simulink model "sim_aut_dual_scen"  (R2025b)
settings: Solver=ode45  StartTime=0.0  StopTime=Tfin  FixedStep=1e-3  MaxStep=1e-2  MinStep=1e-3  RelTol=5e-3
values from neighbouring files (symbols this model uses):
  bp = [-1.25 -1.19897959184 -1.14795918367 -1.09693877551 -1.04591836735 -0.994897959184 -0.94387755102 -0.892857142857 -0.841836734694 -0.790816326531 -0.739795918367 -0.688775510204 ... (50 elements, 1x50)]    [tire_model.mat]
  C1 = 2.7e4    (= 27000)    [main.m]    (also in model.m)
  C2 = 2e4    (= 20000)    [main.m]    (also in model.m)
  Jz = 4000    [main.m]    (also in model.m)
  K = nmpc_design_st2(par,2)    [main.m]
  l1 = 1.2    [main.m]    (also in model.m)
  l2 = 1.6    [main.m]    (also in model.m)
  m = 1575    [main.m]    (also in model.m)
  Np = round(vx_ref*K.Tp/mean(ds))    [main.m]
  pacf = [2550.90487699 2674.70463742 2810.77279096 2960.97362657 3127.55760929 3313.26346728 3521.4532226 3756.29269015 4022.99538347 4328.15571957 4680.20907939 5090.07319782 ... (50 elements, 1x50)]    [tire_model.mat]
  pacr = [2550.90487699 2674.70463742 2810.77279096 2960.97362657 3127.55760929 3313.26346728 3521.4532226 3756.29269015 4022.99538347 4328.15571957 4680.20907939 5090.07319782 ... (50 elements, 1x50)]    [tire_model.mat]
  psi = x(3)    [model.m]
  psir = [atan2(diff(Yr),diff(Xr));0]    [main.m]
  refPoses = [Xr,Yr,psir]    [main.m]
  Ts = 0.05    [main.m]
  ze0 = [X0;Y0;psi0;vx0;vy0;wpsi0]    [main.m]
undefined symbols (not defined in the file or in its folder): aMode, plot_ref, x_o
libraries: autolibsharedcommon x11, autolibshared x5, autolibpowerinfoutils x2, autolibutils x2, sharedtransform x2, simulink x1, drivingscenarioandsensors x1
(part 3 of 4)

== system sim_aut_dual_scen/vehicle/dual-track/Vehicle Body 3DOF Dual Track/Signal Routing/Signal Routing Dual/Moments ==
  MBody : Inport
  Mdrag : Inport  Port=2
  MExt : Inport  Port=3
  Mh : Inport  Port=4
  Bus Creator{1..3,24} (4 alike) : BusCreator  Inputs=3
  Bus Creator7 : BusCreator  Inputs=4
  Demux{,1..3} (4 alike) : Demux  Outputs=3
  Signal Specification{1..11,23} (12 alike) : SignalSpecification  Unit=N*m
  Moments : Outport  VectorParamsAs1DForOutWhenUnconnected=off
  wires:
  Signal Specification11/1 -> Bus Creator2/1  "Mx"
  Demux3/1 -> Signal Specification11/1
  Demux3/3 -> Signal Specification10/1
  Bus Creator2/1 -> Bus Creator7/4  "Hitch"
  Demux3/2 -> Signal Specification9/1
  Signal Specification9/1 -> Bus Creator2/2  "My"
  Mh/1 -> Demux3/1
  Signal Specification10/1 -> Bus Creator2/3  "Mz"
  Signal Specification23/1 -> Bus Creator24/1  "Mx"
  Bus Creator24/1 -> Bus Creator7/1  "Body"
  Signal Specification1/1 -> Bus Creator24/2  "My"
  Signal Specification2/1 -> Bus Creator24/3  "Mz"
  Bus Creator1/1 -> Bus Creator7/2  "Drag"
  Bus Creator7/1 -> Moments/1  "Moments"
  Demux/2 -> Signal Specification1/1
  Demux/1 -> Signal Specification23/1
  Demux/3 -> Signal Specification2/1
  MBody/1 -> Demux/1
  Mdrag/1 -> Demux1/1
  Demux1/3 -> Signal Specification4/1
  Demux1/1 -> Signal Specification5/1
  Demux1/2 -> Signal Specification3/1
  Signal Specification4/1 -> Bus Creator1/3  "Mz"
  Signal Specification3/1 -> Bus Creator1/2  "My"
  Signal Specification5/1 -> Bus Creator1/1  "Mx"
  MExt/1 -> Demux2/1
  Signal Specification7/1 -> Bus Creator3/3  "Mz"
  Signal Specification6/1 -> Bus Creator3/2  "My"
  Bus Creator3/1 -> Bus Creator7/3  "Ext"
  Signal Specification8/1 -> Bus Creator3/1  "Mx"
  Demux2/2 -> Signal Specification6/1
  Demux2/1 -> Signal Specification8/1
  Demux2/3 -> Signal Specification7/1

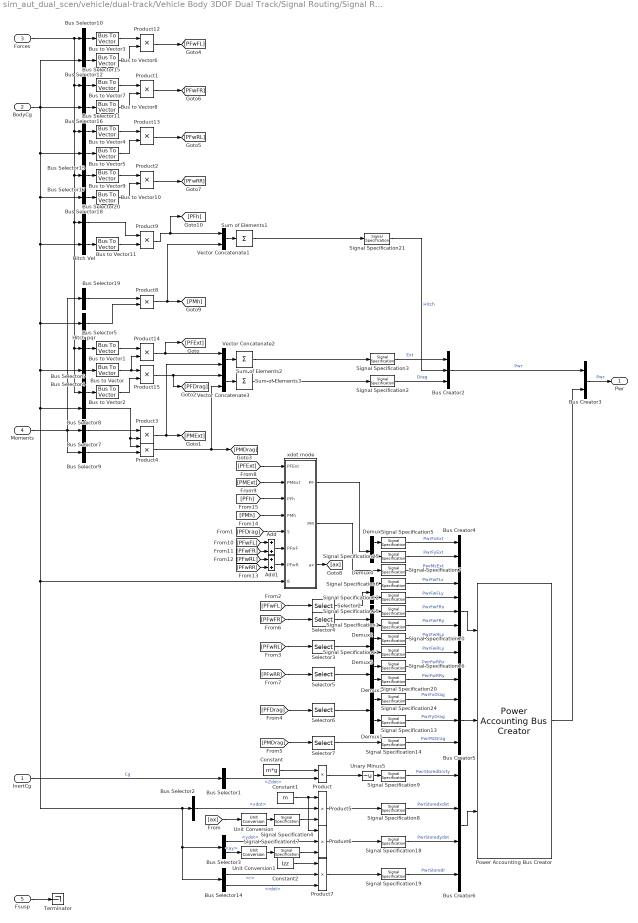
== system sim_aut_dual_scen/vehicle/dual-track/Vehicle Body 3DOF Dual Track/Signal Routing/Signal Routing Dual/Power ==
  InertCg : Inport
  BodyCg : Inport  Port=2
  Forces : Inport  Port=3
  Moments : Inport  Port=4
  Fsusp : Inport  Port=5
  Add : Sum
  Add1 : Sum
  Bus Creator2 : BusCreator  Inputs=3
  Bus Creator3 : BusCreator  Inputs=2
  Bus Creator4 : BusCreator  Inputs=11
  Bus Creator5 : BusCreator  Inputs=3
  Bus Creator6 : BusCreator  Inputs=4
  Bus Selector1 : BusSelector  OutputSignals=Cg.Vel.Zdot
  Bus Selector10 : BusSelector  OutputSignals=FrntAxl.Lft.Fx,FrntAxl.Lft.Fy,FrntAxl.Lft.Fz  OutputAsBus=on
  Bus Selector11 : BusSelector  OutputSignals=RearAxl.Lft.Fx,RearAxl.Lft.Fy,RearAxl.Lft.Fz  OutputAsBus=on
  Bus Selector12 : BusSelector  OutputSignals=FrntAxl.Lft.Vel.xdot,FrntAxl.Lft.Vel.ydot,FrntAxl.Lft.Vel.zdot  OutputAsBus=on
  Bus Selector13 : BusSelector  OutputSignals=RearAxl.Lft.Vel.xdot,RearAxl.Lft.Vel.ydot,RearAxl.Lft.Vel.zdot  OutputAsBus=on
  Bus Selector14 : BusSelector  OutputSignals=Cg.AngVel.r,Cg.AngAcc.rdot
  Bus Selector15 : BusSelector  OutputSignals=FrntAxl.Rght.Fx,FrntAxl.Rght.Fy,FrntAxl.Rght.Fz  OutputAsBus=on
  Bus Selector16 : BusSelector  OutputSignals=FrntAxl.Rght.Vel.xdot,FrntAxl.Rght.Vel.ydot,FrntAxl.Rght.Vel.zdot  OutputAsBus=on
  Bus Selector17 : BusSelector  OutputSignals=RearAxl.Rght.Fx,RearAxl.Rght.Fy,RearAxl.Rght.Fz  OutputAsBus=on
  Bus Selector18 : BusSelector  OutputSignals=RearAxl.Rght.Vel.xdot,RearAxl.Rght.Vel.ydot,RearAxl.Rght.Vel.zdot  OutputAsBus=on
  Bus Selector19 : BusSelector  OutputSignals=Hitch.Mx,Hitch.My,Hitch.Mz  OutputAsBus=on
  Bus Selector2 : BusSelector  OutputSignals=Cg.Vel.xdot
  Bus Selector20 : BusSelector  OutputSignals=Hitch.Fx,Hitch.Fy,Hitch.Fz  OutputAsBus=on
  Bus Selector3 : BusSelector  OutputSignals=Cg.Vel.ydot,Cg.Acc.ay
  Bus Selector4 : BusSelector  OutputSignals=Cg.Vel.xdot,Cg.Vel.ydot,Cg.Vel.zdot  OutputAsBus=on
  Bus Selector5 : BusSelector  OutputSignals=Ext.Fx,Ext.Fy,Ext.Fz  OutputAsBus=on
  Bus Selector6 : BusSelector  OutputSignals=Drag.Fx,Drag.Fy,Drag.Fz  OutputAsBus=on
  Bus Selector7 : BusSelector  OutputSignals=Ext.Mx,Ext.My,Ext.Mz  OutputAsBus=on
  Bus Selector8 : BusSelector  OutputSignals=Cg.AngVel.p,Cg.AngVel.q,Cg.AngVel.r  OutputAsBus=on
  Bus Selector9 : BusSelector  OutputSignals=Drag.Mx,Drag.My,Drag.Mz  OutputAsBus=on
  Bus to Vector{,1..11} (12 alike) : BusToVector
  Constant : Constant  Value=m*g
  Constant1 : Constant  Value=m
  Constant2 : Constant  Value=Izz
  Demux{,1..5} (6 alike) : Demux  Outputs=2
  Hitch Vel : BusSelector  OutputSignals=Hitch.Vel.xdot,Hitch.Vel.ydot,Hitch.Vel.zdot  OutputAsBus=on
  Hitch pqr : BusSelector  OutputSignals=Cg.AngVel.p,Cg.AngVel.q,Cg.AngVel.r  OutputAsBus=on
  Power Accounting Bus Creator : autolibpowerinfoutils/Power Accounting Bus Creator  AssctBlkSelPopup=Parent reference block  RefBlkName='autolibshared/Vehicle Body 3DOF Single Track'  PwrTrnsfrdCheckBox=on  PwrNotTrnsfrdCheckBox=on  PwrStoredCheckBox=on  aMode=aMode
  Product{,1..4,8..9,12..15} (11 alike) : Product
  Product5 : Product  Inputs=3
  Product6 : Product  Inputs=3
  Product7 : Product  Inputs=3
  Selector{2..6} (5 alike) : Selector  InputPortWidth=3  IndexOptions=Index vector (dialog)  Indices=[1 2]  OutputSizes=1
  Selector7 : Selector  InputPortWidth=3  IndexOptions=Index vector (dialog)  Indices=[3]  OutputSizes=1
  Signal Specification{1..3,5..16,18..21,24..25} (21 alike) : SignalSpecification  Unit=W
  Signal Specification17 : SignalSpecification  Unit=m/s^2
  Signal Specification4 : SignalSpecification  Unit=m/s^2
  Sum of Elements1 : Sum  Inputs=+
  Sum of Elements2 : Sum  Inputs=+
  Sum of Elements3 : Sum  Inputs=+
  Terminator : Terminator
  Unary Minus5 : UnaryMinus
  Unit Conversion : UnitConversion
  Unit Conversion1 : UnitConversion
  Vector Concatenate1 : Concatenate
  Vector Concatenate2 : Concatenate
  Vector Concatenate3 : Concatenate
  xdot mode : Subsystem  Variant=on  VariantControlMode=label  LabelModeActiveChoice=1
  Pwr : Outport  VectorParamsAs1DForOutWhenUnconnected=off
  wires:
  [PMh] -> xdot mode/4(PMh)
  [PFh] -> xdot mode/3(PFh)
  Vector Concatenate1/1 -> Sum of Elements1/1
  Forces/1 -> Bus Selector10/1, Bus Selector11/1, Bus Selector5/1, Bus Selector6/1, Bus Selector20/1, Bus Selector17/1, Bus Selector15/1
  BodyCg/1 -> Bus Selector12/1, Bus Selector13/1, Bus Selector4/1, Bus Selector8/1, xdot mode/8(BodyFrm), Bus Selector3/1, Bus Selector14/1, Bus Selector2/1, Hitch pqr/1, Hitch Vel/1, Bus Selector18/1, Bus Selector16/1
  Signal Specification21/1 -> Bus Creator2/2  "Hitch"
  Hitch Vel/1 -> Bus to Vector11/1
  Bus to Vector11/1 -> Product9/2
  Product9/1 -> Vector Concatenate1/1, [PFh]
  Sum of Elements1/1 -> Signal Specification21/1
  Bus Selector20/1 -> Product9/1
  Hitch pqr/1 -> Product8/2
  Bus Selector19/1 -> Product8/1
  Product8/1 -> [PMh], Vector Concatenate1/2
  Signal Specification16/1 -> Bus Creator4/10  "PwrFwRRx"
  [PFwRR] -> Selector5/1
  Signal Specification20/1 -> Bus Creator4/11  "PwrFwRRy"
  Demux3/2 -> Signal Specification20/1
  Selector5/1 -> Demux3/1
  Demux3/1 -> Signal Specification16/1
  [PFwFR] -> Selector4/1
  Signal Specification15/1 -> Bus Creator4/6  "PwrFwFRx"
  Signal Specification1/1 -> Bus Creator4/7  "PwrFwFRy"
  Selector4/1 -> Demux2/1
  Demux2/1 -> Signal Specification15/1
  Demux2/2 -> Signal Specification1/1
  Bus Selector17/1 -> Bus to Vector9/1
  Product2/1 -> [PFwRR]
  Bus Selector18/1 -> Bus to Vector10/1
  Bus to Vector9/1 -> Product2/1
  Bus to Vector10/1 -> Product2/2
  Bus Selector16/1 -> Bus to Vector8/1
  Product1/1 -> [PFwFR]
  Bus Selector15/1 -> Bus to Vector7/1
  Bus to Vector8/1 -> Product1/2
  Bus to Vector7/1 -> Product1/1
  Fsusp/1 -> Terminator/1
  Product4/1 -> [PMDrag], Vector Concatenate3/2
  Power Accounting Bus Creator/1 -> Bus Creator3/2
  Unit Conversion/1 -> Signal Specification4/1
  Demux4/2 -> Signal Specification12/1
  Constant/1 -> Product/1
  Product6/1 -> Signal Specification18/1
  Demux/1 -> Signal Specification5/1
  Bus to Vector5/1 -> Product13/2
  Product/1 -> Unary Minus5/1
  Signal Specification25/1 -> Bus Creator4/2  "PwrFyExt"
  Constant1/1 -> Product6/1, Product5/1
  Bus to Vector/1 -> Product14/2, Product15/1
  Signal Specification5/1 -> Bus Creator4/1  "PwrFxExt"
  Demux5/1 -> Signal Specification10/1
  Signal Specification24/1 -> Bus Creator5/1  "PwrFxDrag"
  Unary Minus5/1 -> Signal Specification9/1
  Product12/1 -> [PFwFL]
  Demux1/1 -> Signal Specification24/1
  Demux4/1 -> Signal Specification6/1
  Selector3/1 -> Demux5/1
  Bus Selector9/1 -> Product4/2
  Signal Specification17/1 -> Product6/3
  Demux5/2 -> Signal Specification11/1
  Selector2/1 -> Demux4/1
  Signal Specification12/1 -> Bus Creator4/5  "PwrFwFLy"
  Unit Conversion1/1 -> Signal Specification17/1
  Signal Specification10/1 -> Bus Creator4/8  "PwrFwRLx"
  Bus Selector8/1 -> Product3/2, Product4/1
  Signal Specification2/1 -> Bus Creator2/3  "Drag"
  Bus Selector7/1 -> Product3/1
  xdot mode/2(PM) -> Signal Specification7/1
  Signal Specification11/1 -> Bus Creator4/9  "PwrFwRLy"
  Signal Specification9/1 -> Bus Creator6/1  "PwrStoredGrvty"
  Bus to Vector4/1 -> Product13/1
  Bus Creator3/1 -> Pwr/1  "Pwr"
  Signal Specification6/1 -> Bus Creator4/4  "PwrFwFLx"
  Bus Selector12/1 -> Bus to Vector6/1
  Selector6/1 -> Demux1/1
  [PFDrag] -> Selector6/1
  Signal Specification13/1 -> Bus Creator5/2  "PwrFyDrag"
  Bus to Vector3/1 -> Product12/1
  Bus Selector4/1 -> Bus to Vector/1
  Signal Specification7/1 -> Bus Creator4/3  "PwrMzExt"
  [PFwFL] -> Selector2/1
  [ax] -> Unit Conversion/1
  Signal Specification14/1 -> Bus Creator5/3  "PwrMzDrag"
  Demux1/2 -> Signal Specification13/1
  [PMDrag] -> Selector7/1
  Bus to Vector6/1 -> Product12/2
  Bus Selector10/1 -> Bus to Vector3/1
  xdot mode/1(PF) -> Demux/1
  Bus Selector14/1 -> Product7/2  "<r>"
  Bus Selector14/2 -> Product7/3  "<rdot>"
  Signal Specification18/1 -> Bus Creator6/3  "PwrStoredydot"
  Bus Selector3/2 -> Unit Conversion1/1  "<ay>"
  Vector Concatenate3/1 -> Sum of Elements3/1
  Bus Selector2/1 -> Product5/2  "<xdot>"
  Signal Specification19/1 -> Bus Creator6/4  "PwrStoredr"
  Vector Concatenate2/1 -> Sum of Elements2/1
  Moments/1 -> Bus Selector9/1, Bus Selector19/1, Bus Selector7/1
  Bus Selector13/1 -> Bus to Vector5/1
  Bus to Vector2/1 -> Product15/2
  Sum of Elements2/1 -> Signal Specification3/1
  Constant2/1 -> Product7/1
  Bus Selector3/1 -> Product6/2  "<ydot>"
  Product7/1 -> Signal Specification19/1
  Product13/1 -> [PFwRL]
  Selector7/1 -> Signal Specification14/1
  Demux/2 -> Signal Specification25/1
  [PFwRL] -> Selector3/1
  Signal Specification8/1 -> Bus Creator6/2  "PwrStoredxdot"
  Bus Selector6/1 -> Bus to Vector2/1
  Bus to Vector1/1 -> Product14/1
  Sum of Elements3/1 -> Signal Specification2/1
  InertCg/1 -> Bus Selector1/1  "Cg"
  Bus Selector11/1 -> Bus to Vector4/1
  Product3/1 -> Vector Concatenate2/2, [PMExt]
  Bus Selector1/1 -> Product/2  "<Zdot>"
  Signal Specification4/1 -> Product5/3
  Bus Selector5/1 -> Bus to Vector1/1
  Product14/1 -> Vector Concatenate2/1, [PFExt]
  Bus Creator2/1 -> Bus Creator3/1  "Pwr"
  Product15/1 -> Vector Concatenate3/1, [PFDrag]
  Signal Specification3/1 -> Bus Creator2/1  "Ext"
  Add/1 -> xdot mode/6(PFwF)
  [PFDrag] -> xdot mode/5(PFDrag)
  [PFExt] -> xdot mode/1(PFExt)
  [PMExt] -> xdot mode/2(PMExt)
  [PFwFL] -> Add/1
  [PFwFR] -> Add/2
  [PFwRL] -> Add1/1
  [PFwRR] -> Add1/2
  Add1/1 -> xdot mode/7(PFwR)
  Bus Creator5/1 -> Power Accounting Bus Creator/2
  Bus Creator4/1 -> Power Accounting Bus Creator/1
  Bus Creator6/1 -> Power Accounting Bus Creator/3
  Product5/1 -> Signal Specification8/1
  xdot mode/3(ax) -> [ax]

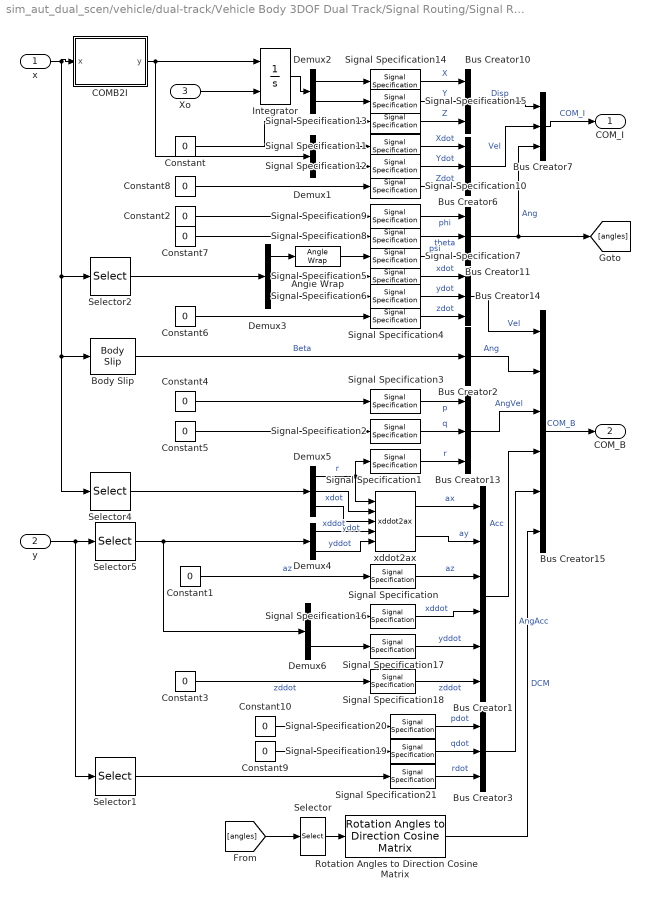
== system sim_aut_dual_scen/vehicle/dual-track/Vehicle Body 3DOF Dual Track/Signal Routing/Signal Routing Dual/state2bus ==
  x : Inport
  y : Inport  Port=2
  Xo : Inport  Port=3
  Angle Wrap : autolibshared/Vehicle Body 3DOF Single Track/Signal Routing/Signal Routing/state2bus/Angle Wrap  SystemSampleTime=-1  VariantControl=Variant1  LabelModeActiveChoice=None  VariantActivationTime=update diagram  EmptyChoice=off  PassThrough=off  PassThroughVariantControl=(default)  EmptyChoiceVariantControl=(default)  AllowFlexibleInterface=on  Latency=0  AutoFrameSizeCalculation=off
  Body Slip : autolibshared/Vehicle Body 3DOF Single Track/Signal Routing/Signal Routing/state2bus/Body Slip  SystemSampleTime=-1  VariantActivationTime=update diagram  EmptyChoice=off  PassThrough=off  PassThroughVariantControl=(default)  EmptyChoiceVariantControl=(default)  AllowFlexibleInterface=on  Latency=0  AutoFrameSizeCalculation=off
  Bus Creator1 : BusCreator  Inputs=6
  Bus Creator{3,6..7,10..11,13..14} (7 alike) : BusCreator  Inputs=3
  Bus Creator15 : BusCreator  Inputs=6
  Bus Creator2 : BusCreator  Inputs=1
  COMB2I : MATLAB Function  TreatAsAtomicUnit=on
  Constant{,1..10} (11 alike) : Constant  Value=0
  Demux{1..2,4,6} (4 alike) : Demux  Outputs=2
  Demux3 : Demux  Outputs=3
  Demux5 : Demux  Outputs=3
  Integrator : Integrator  InitialConditionSource=external
  Rotation Angles to Direction Cosine Matrix : sharedtransform/Rotation Angles to Direction Cosine Matrix  rotationOrder=ZYX  aMode=aMode
  Selector : Selector  InputPortWidth=3  IndexOptions=Index vector (dialog)  Indices=[3 2 1]  OutputSizes=1
  Selector1 : Selector  IndexOptions=Index vector (dialog)  Indices=[3]  OutputSizes=1
  Selector2 : Selector  IndexOptions=Index vector (dialog)  Indices=[3,1,2]  OutputSizes=1
  Selector4 : Selector  IndexOptions=Index vector (dialog)  Indices=[4,1,2]  OutputSizes=1
  Selector5 : Selector  IndexOptions=Index vector (dialog)  Indices=[1,2]  OutputSizes=1
  Signal Specification : SignalSpecification  Unit=gn
  Signal Specification1 : SignalSpecification  Unit=rad/s
  Signal Specification{4..6,10..12} (6 alike) : SignalSpecification  Unit=m/s
  Signal Specification13 : SignalSpecification  Unit=m
  Signal Specification14 : SignalSpecification  Unit=m
  Signal Specification15 : SignalSpecification  Unit=m
  Signal Specification16 : SignalSpecification  Unit=m/s^2
  Signal Specification17 : SignalSpecification  Unit=m/s^2
  Signal Specification18 : SignalSpecification  Unit=m/s^2
  Signal Specification19 : SignalSpecification  Unit=rad/s^2
  Signal Specification2 : SignalSpecification  Unit=rad/s
  Signal Specification20 : SignalSpecification  Unit=rad/s^2
  Signal Specification21 : SignalSpecification  Unit=rad/s^2
  Signal Specification3 : SignalSpecification  Unit=rad/s
  Signal Specification7 : SignalSpecification  Unit=rad
  Signal Specification8 : SignalSpecification  Unit=rad
  Signal Specification9 : SignalSpecification  Unit=rad
  xddot2ax : autolibshared/Vehicle Body 3DOF Single Track/Signal Routing/Signal Routing/state2bus/xddot2ax  SystemSampleTime=-1  VariantActivationTime=update diagram  EmptyChoice=off  PassThrough=off  PassThroughVariantControl=(default)  EmptyChoiceVariantControl=(default)  AllowFlexibleInterface=on  Latency=0  AutoFrameSizeCalculation=off
  COM_I : Outport  VectorParamsAs1DForOutWhenUnconnected=off
  COM_B : Outport  Port=2  VectorParamsAs1DForOutWhenUnconnected=off
  wires:
  Rotation Angles to Direction Cosine Matrix/1 -> Bus Creator15/6  "DCM"
  Selector/1 -> Rotation Angles to Direction Cosine Matrix/1
  [angles] -> Selector/1
  Angle Wrap/1 -> Signal Specification7/1
  Constant10/1 -> Signal Specification20/1
  Bus Creator3/1 -> Bus Creator15/5  "AngAcc"
  Constant9/1 -> Signal Specification19/1
  Signal Specification20/1 -> Bus Creator3/1  "pdot"
  Selector1/1 -> Signal Specification21/1
  Signal Specification19/1 -> Bus Creator3/2  "qdot"
  Signal Specification21/1 -> Bus Creator3/3  "rdot"
  Xo/1 -> Integrator/2
  Bus Creator2/1 -> Bus Creator15/2  "Ang"
  Body Slip/1 -> Bus Creator2/1  "Beta"
  Demux6/2 -> Signal Specification17/1
  Demux6/1 -> Signal Specification16/1
  Signal Specification16/1 -> Bus Creator1/4  "xddot"
  Signal Specification18/1 -> Bus Creator1/6  "zddot"
  Signal Specification17/1 -> Bus Creator1/5  "yddot"
  Bus Creator1/1 -> Bus Creator15/4  "Acc"
  xddot2ax/1 -> Bus Creator1/1  "ax"
  Demux5/1 -> xddot2ax/1, Signal Specification1/1  "r"
  xddot2ax/2 -> Bus Creator1/2  "ay"
  Selector5/1 -> Demux6/1, Demux4/1
  Demux4/2 -> xddot2ax/5  "yddot"
  Constant3/1 -> Signal Specification18/1  "zddot"
  Signal Specification/1 -> Bus Creator1/3  "az"
  Demux5/3 -> xddot2ax/3  "ydot"
  Constant1/1 -> Signal Specification/1  "az"
  Selector4/1 -> Demux5/1
  Demux4/1 -> xddot2ax/4  "xddot"
  Demux5/2 -> xddot2ax/2  "xdot"
  y/1 -> Selector5/1, Selector1/1
  Demux2/1 -> Signal Specification14/1
  Demux2/2 -> Signal Specification15/1
  Constant/1 -> Signal Specification13/1
  Demux1/1 -> Signal Specification11/1
  Demux1/2 -> Signal Specification12/1
  Constant8/1 -> Signal Specification10/1
  Constant2/1 -> Signal Specification9/1
  Constant7/1 -> Signal Specification8/1
  Demux3/1 -> Angle Wrap/1
  Demux3/3 -> Signal Specification6/1
  Demux3/2 -> Signal Specification5/1
  Constant6/1 -> Signal Specification4/1
  Constant4/1 -> Signal Specification3/1
  Constant5/1 -> Signal Specification2/1
  Signal Specification1/1 -> Bus Creator13/3  "r"
  x/1 -> Selector4/1, Body Slip/1, Selector2/1, COMB2I/1(x)
  Signal Specification10/1 -> Bus Creator6/3  "Zdot"
  Signal Specification4/1 -> Bus Creator14/3  "zdot"
  Signal Specification11/1 -> Bus Creator6/1  "Xdot"
  Signal Specification15/1 -> Bus Creator10/2  "Y"
  Bus Creator13/1 -> Bus Creator15/3  "AngVel"
  Signal Specification13/1 -> Bus Creator10/3  "Z"
  Signal Specification14/1 -> Bus Creator10/1  "X"
  Signal Specification9/1 -> Bus Creator11/1  "phi"
  Bus Creator7/1 -> COM_I/1  "COM_I"
  Signal Specification3/1 -> Bus Creator13/1  "p"
  Bus Creator14/1 -> Bus Creator15/1  "Vel"
  Bus Creator6/1 -> Bus Creator7/2  "Vel"
  Bus Creator10/1 -> Bus Creator7/1  "Disp"
  Signal Specification8/1 -> Bus Creator11/2  "theta"
  Selector2/1 -> Demux3/1
  Signal Specification12/1 -> Bus Creator6/2  "Ydot"
  Signal Specification2/1 -> Bus Creator13/2  "q"
  Bus Creator15/1 -> COM_B/1  "COM_B"
  Signal Specification5/1 -> Bus Creator14/1  "xdot"
  Bus Creator11/1 -> Bus Creator7/3, [angles]  "Ang"
  Signal Specification6/1 -> Bus Creator14/2  "ydot"
  Integrator/1 -> Demux2/1
  COMB2I/1(y) -> Integrator/1, Demux1/1
  Signal Specification7/1 -> Bus Creator11/3  "psi"

== system sim_aut_dual_scen/vehicle/dual-track/Vehicle Body 3DOF Dual Track/sigma/sigma/relaxation front ==
  alpha : Inport
  V : Inport  Port=2
  sigma : Inport  Port=3
  Product1 : Product  Inputs=**/  InputSameDT=on  RndMeth=Zero  SaturateOnIntegerOverflow=on  OutDataTypeStr=Inherit: Same as first input
  Sum : Sum  Inputs=-+|  InputSameDT=on  SaturateOnIntegerOverflow=on  OutDataTypeStr=Inherit: Same as first input
  lateral : Integrator
  alpha_sig : Outport  VectorParamsAs1DForOutWhenUnconnected=off
  wires:
  lateral/1 -> alpha_sig/1, Sum/1
  sigma/1 -> Product1/3
  Sum/1 -> Product1/1
  Product1/1 -> lateral/1
  V/1 -> Product1/2
  alpha/1 -> Sum/2

== system sim_aut_dual_scen/vehicle/dual-track/Vehicle Body 3DOF Dual Track/sigma/sigma/relaxation rear ==
  alpha : Inport
  V : Inport  Port=2
  sigma : Inport  Port=3
  Product1 : Product  Inputs=**/  InputSameDT=on  RndMeth=Zero  SaturateOnIntegerOverflow=on  OutDataTypeStr=Inherit: Same as first input
  Sum : Sum  Inputs=-+|  InputSameDT=on  SaturateOnIntegerOverflow=on  OutDataTypeStr=Inherit: Same as first input
  lateral : Integrator
  alpha_sig : Outport  VectorParamsAs1DForOutWhenUnconnected=off
  wires:
  alpha/1 -> Sum/2
  V/1 -> Product1/2
  Product1/1 -> lateral/1
  Sum/1 -> Product1/1
  sigma/1 -> Product1/3
  lateral/1 -> alpha_sig/1, Sum/1

== system sim_aut_dual_scen/vehicle/dual-track/Vehicle Body 3DOF Dual Track/sigma/sigma dual/relaxation ==
  alpha : Inport
  V : Inport  Port=2
  sigma : Inport  Port=3
  Product1 : Product  Inputs=**/  InputSameDT=on  RndMeth=Zero  SaturateOnIntegerOverflow=on  OutDataTypeStr=Inherit: Same as first input
  Sum : Sum  Inputs=-+|  InputSameDT=on  SaturateOnIntegerOverflow=on  OutDataTypeStr=Inherit: Same as first input
  lateral : Integrator
  alpha_sig : Outport  VectorParamsAs1DForOutWhenUnconnected=off
  wires:
  alpha/1 -> Sum/2
  V/1 -> Product1/2
  Product1/1 -> lateral/1
  Sum/1 -> Product1/1
  sigma/1 -> Product1/3
  lateral/1 -> Sum/1, alpha_sig/1

== system sim_aut_dual_scen/vehicle/dual-track/Vehicle Body 3DOF Dual Track/sigma1/sigma/relaxation front ==
  alpha : Inport
  V : Inport  Port=2
  sigma : Inport  Port=3
  Product1 : Product  Inputs=**/  InputSameDT=on  RndMeth=Zero  SaturateOnIntegerOverflow=on  OutDataTypeStr=Inherit: Same as first input
  Sum : Sum  Inputs=-+|  InputSameDT=on  SaturateOnIntegerOverflow=on  OutDataTypeStr=Inherit: Same as first input
  lateral : Integrator
  alpha_sig : Outport  VectorParamsAs1DForOutWhenUnconnected=off
  wires:
  alpha/1 -> Sum/2
  V/1 -> Product1/2
  Product1/1 -> lateral/1
  Sum/1 -> Product1/1
  sigma/1 -> Product1/3
  lateral/1 -> Sum/1, alpha_sig/1

== system sim_aut_dual_scen/vehicle/dual-track/Vehicle Body 3DOF Dual Track/sigma1/sigma/relaxation rear ==
  alpha : Inport
  V : Inport  Port=2
  sigma : Inport  Port=3
  Product1 : Product  Inputs=**/  InputSameDT=on  RndMeth=Zero  SaturateOnIntegerOverflow=on  OutDataTypeStr=Inherit: Same as first input
  Sum : Sum  Inputs=-+|  InputSameDT=on  SaturateOnIntegerOverflow=on  OutDataTypeStr=Inherit: Same as first input
  lateral : Integrator
  alpha_sig : Outport  VectorParamsAs1DForOutWhenUnconnected=off
  wires:
  lateral/1 -> Sum/1, alpha_sig/1
  sigma/1 -> Product1/3
  Sum/1 -> Product1/1
  Product1/1 -> lateral/1
  V/1 -> Product1/2
  alpha/1 -> Sum/2

== system sim_aut_dual_scen/vehicle/dual-track/Vehicle Body 3DOF Dual Track/sigma1/sigma dual/relaxation ==
  alpha : Inport
  alpha_sig : Outport  VectorParamsAs1DForOutWhenUnconnected=off
  wires:
  alpha/1 -> alpha_sig/1

== system sim_aut_dual_scen/vehicle/dual-track/Vehicle Body 3DOF Dual Track/Signal Routing/Signal Routing/Lateral 3DOF/Hard Point Coordinate Transform Geometric ==
  InertFrmCg : Inport
  BdyFrmCg : Inport  Port=2
  Hard Point Coordinate Transform External Displacement Beta : autolibsharedcommon/Hard Point Coordinate Transform External Displacement Beta  xdot_tol=xdot_tol  aMode=aMode
  Vector Concatenate : Concatenate  NumInputs=3
  latOff : Constant  Value=latOff
  longOff : Constant  Value=longOff
  vertOff : Constant  Value=vertOff
  Inert : Outport  VectorParamsAs1DForOutWhenUnconnected=off
  Body : Outport  Port=2  VectorParamsAs1DForOutWhenUnconnected=off
  wires:
  latOff/1 -> Vector Concatenate/2
  longOff/1 -> Vector Concatenate/1
  vertOff/1 -> Vector Concatenate/3
  Hard Point Coordinate Transform External Displacement Beta/1 -> Inert/1
  BdyFrmCg/1 -> Hard Point Coordinate Transform External Displacement Beta/2
  Vector Concatenate/1 -> Hard Point Coordinate Transform External Displacement Beta/3
  Hard Point Coordinate Transform External Displacement Beta/2 -> Body/1
  InertFrmCg/1 -> Hard Point Coordinate Transform External Displacement Beta/1

== system sim_aut_dual_scen/vehicle/dual-track/Vehicle Body 3DOF Dual Track/Signal Routing/Signal Routing/Lateral 3DOF/Hitch Coordinate Transform ==
  InertFrmCg : Inport
  BodyFrmCg : Inport  Port=2
  Constant : Constant  Value=dh
  Constant2 : Constant  Value=h
  Constant3 : Constant  Value=hh
  Constant4 : Constant  Value=0
  Hard Point Coordinate Transform External Displacement : autolibsharedcommon/Hard Point Coordinate Transform External Displacement  aMode=aMode
  Sum : Sum  Inputs=|+-
  Unary Minus2 : UnaryMinus
  Vector Concatenate : Concatenate  NumInputs=3
  Inert : Outport
  Body : Outport  Port=2
  wires:
  Constant4/1 -> Vector Concatenate/2
  Sum/1 -> Vector Concatenate/3
  Constant3/1 -> Sum/2
  Constant2/1 -> Sum/1
  Unary Minus2/1 -> Vector Concatenate/1
  Hard Point Coordinate Transform External Displacement/2 -> Body/1
  Hard Point Coordinate Transform External Displacement/1 -> Inert/1
  Vector Concatenate/1 -> Hard Point Coordinate Transform External Displacement/3
  Constant/1 -> Unary Minus2/1
  InertFrmCg/1 -> Hard Point Coordinate Transform External Displacement/1
  BodyFrmCg/1 -> Hard Point Coordinate Transform External Displacement/2

== system sim_aut_dual_scen/vehicle/dual-track/Vehicle Body 3DOF Dual Track/Signal Routing/Signal Routing/Power/xdot mode ==
  note: 1) Add Subsystem or Model blocks as valid variant choices.
      | 2) You cannot connect blocks at this level. At simulation, connectivity is automatically
      | determined, based on the active variant and port name matching.
  PFExt : Inport
  PMExt : Inport  Port=2
  PFh : Inport  Port=3
  PMh : Inport  Port=4
  PFDrag : Inport  Port=5
  PFwF : Inport  Port=6
  PFwR : Inport  Port=7
  BodyFrm : Inport  Port=8
  FxIn : Subsystem  VariantControl=1
  xdotin : Subsystem  VariantControl=0
  PF : Outport  VectorParamsAs1DForOutWhenUnconnected=off
  PM : Outport  Port=2  VectorParamsAs1DForOutWhenUnconnected=off
  ax : Outport  Port=3  VectorParamsAs1DForOutWhenUnconnected=off

== system sim_aut_dual_scen/vehicle/dual-track/Vehicle Body 3DOF Dual Track/Signal Routing/Signal Routing/state2bus/Angle Wrap ==
  "u " : Inport
  None : Subsystem  VariantControl=None
  Wrap : autolibutils/Wrap  VariantControl=Wrap  aMode=aMode
  " y" : Outport  VectorParamsAs1DForOutWhenUnconnected=off

== system sim_aut_dual_scen/vehicle/dual-track/Vehicle Body 3DOF Dual Track/Signal Routing/Signal Routing/state2bus/Body Slip ==
  x : Inport
  Demux7 : Demux  Outputs=2
  Divide : Product  Inputs=*/
  Selector1 : Selector  IndexOptions=Index vector (dialog)  Indices=[2,1]  OutputSizes=1
  Signal Specification9 : SignalSpecification  Unit=rad
  Trigonometric Function : Trigonometry  Operator=atan  OutputSignalType=real
  div0protect - abs poly : autolibutils/div0protect - abs poly  thresh=xdot_tol  aMode=aMode
  Beta : Outport  VectorParamsAs1DForOutWhenUnconnected=off
  wires:
  Signal Specification9/1 -> Beta/1
  Divide/1 -> Trigonometric Function/1
  Trigonometric Function/1 -> Signal Specification9/1  "Beta"
  Selector1/1 -> Demux7/1
  x/1 -> Selector1/1
  Demux7/1 -> Divide/1
  div0protect - abs poly/1 -> Divide/2
  Demux7/2 -> div0protect - abs poly/1

== system sim_aut_dual_scen/vehicle/dual-track/Vehicle Body 3DOF Dual Track/Signal Routing/Signal Routing/state2bus/xddot2ax ==
  r : Inport
  xdot : Inport  Port=2
  ydot : Inport  Port=3
  xddot : Inport  Port=4
  yddot : Inport  Port=5
  Divide : Product  Inputs=**
  Divide1 : Product  Inputs=**
  Sum of Elements : Sum
  Sum of Elements1 : Sum  Inputs=-+
  m^22gn : Subsystem
  ax : Outport  Unit=gn  VectorParamsAs1DForOutWhenUnconnected=off
  ay : Outport  Port=2  Unit=gn  VectorParamsAs1DForOutWhenUnconnected=off
  wires:
  xddot/1 -> Sum of Elements1/2
  xdot/1 -> Divide/1
  ydot/1 -> Divide1/2
  r/1 -> Divide/2, Divide1/1
  Divide/1 -> Sum of Elements/2
  Divide1/1 -> Sum of Elements1/1
  yddot/1 -> Sum of Elements/1
  Sum of Elements/1 -> m^22gn/1(ay)  "ay"
  Sum of Elements1/1 -> m^22gn/2(ax)  "ax"
  m^22gn/2(ax_g) -> ax/1
  m^22gn/1(ay_g) -> ay/1

== system sim_aut_dual_scen/vehicle/dual-track/Vehicle Body 3DOF Dual Track/Signal Routing/Signal Routing Dual/Lateral 3DOF/Hard Point Coordinate Transform Front Left ==
  InertFrmCg : Inport
  BdyFrmCg : Inport  Port=2
  Gain : Gain  Gain=-1/2
  Hard Point Coordinate Transform External Displacement : autolibsharedcommon/Hard Point Coordinate Transform External Displacement  aMode=aMode
  Selector : Selector  InputPortWidth=2  IndexOptions=Index vector (dialog)  Indices=[1]  OutputSizes=1
  Subtract : Sum  Inputs=+-
  Vector Concatenate : Concatenate  NumInputs=3
  a : Constant  Value=a
  d : Constant  Value=d
  h : Constant  Value=h
  w : Constant  Value=w
  Inert : Outport  VectorParamsAs1DForOutWhenUnconnected=off
  Body : Outport  Port=2  VectorParamsAs1DForOutWhenUnconnected=off
  wires:
  Subtract/1 -> Vector Concatenate/2
  d/1 -> Subtract/2
  InertFrmCg/1 -> Hard Point Coordinate Transform External Displacement/1
  w/1 -> Selector/1
  Gain/1 -> Subtract/1
  a/1 -> Vector Concatenate/1
  Hard Point Coordinate Transform External Displacement/2 -> Body/1
  Vector Concatenate/1 -> Hard Point Coordinate Transform External Displacement/3
  h/1 -> Vector Concatenate/3
  BdyFrmCg/1 -> Hard Point Coordinate Transform External Displacement/2
  Hard Point Coordinate Transform External Displacement/1 -> Inert/1
  Selector/1 -> Gain/1

== system sim_aut_dual_scen/vehicle/dual-track/Vehicle Body 3DOF Dual Track/Signal Routing/Signal Routing Dual/Lateral 3DOF/Hard Point Coordinate Transform Front Right ==
  InertFrmCg : Inport
  BdyFrmCg : Inport  Port=2
  Gain : Gain  Gain=1/2
  Hard Point Coordinate Transform External Displacement : autolibsharedcommon/Hard Point Coordinate Transform External Displacement  aMode=aMode
  Selector : Selector  InputPortWidth=2  IndexOptions=Index vector (dialog)  Indices=[1]  OutputSizes=1
  Subtract : Sum  Inputs=+-
  Vector Concatenate : Concatenate  NumInputs=3
  a : Constant  Value=a
  d : Constant  Value=d
  h : Constant  Value=h
  w : Constant  Value=w
  Inert : Outport  VectorParamsAs1DForOutWhenUnconnected=off
  Body : Outport  Port=2  VectorParamsAs1DForOutWhenUnconnected=off
  wires:
  Subtract/1 -> Vector Concatenate/2
  a/1 -> Vector Concatenate/1
  Selector/1 -> Gain/1
  h/1 -> Vector Concatenate/3
  w/1 -> Selector/1
  d/1 -> Subtract/2
  Gain/1 -> Subtract/1
  Hard Point Coordinate Transform External Displacement/1 -> Inert/1
  BdyFrmCg/1 -> Hard Point Coordinate Transform External Displacement/2
  Vector Concatenate/1 -> Hard Point Coordinate Transform External Displacement/3
  Hard Point Coordinate Transform External Displacement/2 -> Body/1
  InertFrmCg/1 -> Hard Point Coordinate Transform External Displacement/1

== system sim_aut_dual_scen/vehicle/dual-track/Vehicle Body 3DOF Dual Track/Signal Routing/Signal Routing Dual/Lateral 3DOF/Hard Point Coordinate Transform Geometric ==
  InertFrmCg : Inport
  BdyFrmCg : Inport  Port=2
  Hard Point Coordinate Transform External Displacement Beta : autolibsharedcommon/Hard Point Coordinate Transform External Displacement Beta  xdot_tol=xdot_tol  aMode=aMode
  Vector Concatenate : Concatenate  NumInputs=3
  latOff : Constant  Value=latOff
  longOff : Constant  Value=longOff
  vertOff : Constant  Value=vertOff
  Inert : Outport  VectorParamsAs1DForOutWhenUnconnected=off
  Body : Outport  Port=2  VectorParamsAs1DForOutWhenUnconnected=off
  wires:
  InertFrmCg/1 -> Hard Point Coordinate Transform External Displacement Beta/1
  Hard Point Coordinate Transform External Displacement Beta/2 -> Body/1
  Vector Concatenate/1 -> Hard Point Coordinate Transform External Displacement Beta/3
  BdyFrmCg/1 -> Hard Point Coordinate Transform External Displacement Beta/2
  Hard Point Coordinate Transform External Displacement Beta/1 -> Inert/1
  vertOff/1 -> Vector Concatenate/3
  longOff/1 -> Vector Concatenate/1
  latOff/1 -> Vector Concatenate/2

== system sim_aut_dual_scen/vehicle/dual-track/Vehicle Body 3DOF Dual Track/Signal Routing/Signal Routing Dual/Lateral 3DOF/Hard Point Coordinate Transform Rear Left ==
  InertFrmCg : Inport
  BdyFrmCg : Inport  Port=2
  Gain : Gain  Gain=-1/2
  Hard Point Coordinate Transform External Displacement : autolibsharedcommon/Hard Point Coordinate Transform External Displacement  aMode=aMode
  Selector : Selector  InputPortWidth=2  IndexOptions=Index vector (dialog)  Indices=[2]  OutputSizes=1
  Subtract : Sum  Inputs=+-
  Vector Concatenate : Concatenate  NumInputs=3
  b : Constant  Value=-b
  d : Constant  Value=d
  h : Constant  Value=h
  w : Constant  Value=w
  Inert : Outport  VectorParamsAs1DForOutWhenUnconnected=off
  Body : Outport  Port=2  VectorParamsAs1DForOutWhenUnconnected=off
  wires:
  Gain/1 -> Subtract/1
  Subtract/1 -> Vector Concatenate/2
  w/1 -> Selector/1
  d/1 -> Subtract/2
  Selector/1 -> Gain/1
  b/1 -> Vector Concatenate/1
  h/1 -> Vector Concatenate/3
  InertFrmCg/1 -> Hard Point Coordinate Transform External Displacement/1
  Hard Point Coordinate Transform External Displacement/2 -> Body/1
  Vector Concatenate/1 -> Hard Point Coordinate Transform External Displacement/3
  BdyFrmCg/1 -> Hard Point Coordinate Transform External Displacement/2
  Hard Point Coordinate Transform External Displacement/1 -> Inert/1

== system sim_aut_dual_scen/vehicle/dual-track/Vehicle Body 3DOF Dual Track/Signal Routing/Signal Routing Dual/Lateral 3DOF/Hard Point Coordinate Transform Rear Right ==
  InertFrmCg : Inport
  BdyFrmCg : Inport  Port=2
  Gain : Gain  Gain=1/2
  Hard Point Coordinate Transform External Displacement : autolibsharedcommon/Hard Point Coordinate Transform External Displacement  aMode=aMode
  Selector : Selector  InputPortWidth=2  IndexOptions=Index vector (dialog)  Indices=[2]  OutputSizes=1
  Subtract : Sum  Inputs=+-
  Vector Concatenate : Concatenate  NumInputs=3
  b : Constant  Value=-b
  d : Constant  Value=d
  h : Constant  Value=h
  w : Constant  Value=w
  Inert : Outport  VectorParamsAs1DForOutWhenUnconnected=off
  Body : Outport  Port=2  VectorParamsAs1DForOutWhenUnconnected=off
  wires:
  Gain/1 -> Subtract/1
  Subtract/1 -> Vector Concatenate/2
  w/1 -> Selector/1
  d/1 -> Subtract/2
  Selector/1 -> Gain/1
  b/1 -> Vector Concatenate/1
  h/1 -> Vector Concatenate/3
  Hard Point Coordinate Transform External Displacement/1 -> Inert/1
  BdyFrmCg/1 -> Hard Point Coordinate Transform External Displacement/2
  Vector Concatenate/1 -> Hard Point Coordinate Transform External Displacement/3
  Hard Point Coordinate Transform External Displacement/2 -> Body/1
  InertFrmCg/1 -> Hard Point Coordinate Transform External Displacement/1

== system sim_aut_dual_scen/vehicle/dual-track/Vehicle Body 3DOF Dual Track/Signal Routing/Signal Routing Dual/Lateral 3DOF/Hitch Coordinate Transform ==
  InertFrmCg : Inport
  BodyFrmCg : Inport  Port=2
  Constant : Constant  Value=dh
  Constant1 : Constant  Value=d
  Constant2 : Constant  Value=h
  Constant3 : Constant  Value=hh
  Constant4 : Constant  Value=hl
  Hard Point Coordinate Transform External Displacement : autolibsharedcommon/Hard Point Coordinate Transform External Displacement  aMode=aMode
  Sum : Sum  Inputs=|+-
  Sum1 : Sum  Inputs=|+-
  Unary Minus2 : UnaryMinus
  Vector Concatenate : Concatenate  NumInputs=3
  Inert : Outport
  Body : Outport  Port=2
  wires:
  Constant1/1 -> Sum1/2
  Unary Minus2/1 -> Vector Concatenate/1
  Constant/1 -> Unary Minus2/1
  Sum/1 -> Vector Concatenate/3
  Constant4/1 -> Sum1/1
  Sum1/1 -> Vector Concatenate/2
  Constant3/1 -> Sum/2
  Constant2/1 -> Sum/1
  BodyFrmCg/1 -> Hard Point Coordinate Transform External Displacement/2
  InertFrmCg/1 -> Hard Point Coordinate Transform External Displacement/1
  Vector Concatenate/1 -> Hard Point Coordinate Transform External Displacement/3
  Hard Point Coordinate Transform External Displacement/1 -> Inert/1
  Hard Point Coordinate Transform External Displacement/2 -> Body/1

== system sim_aut_dual_scen/vehicle/dual-track/Vehicle Body 3DOF Dual Track/Signal Routing/Signal Routing Dual/Power/xdot mode ==
  note: 1) Add Subsystem or Model blocks as valid variant choices.
      | 2) You cannot connect blocks at this level. At simulation, connectivity is automatically
      | determined, based on the active variant and port name matching.
  PFExt : Inport
  PMExt : Inport  Port=2
  PFh : Inport  Port=3
  PMh : Inport  Port=4
  PFDrag : Inport  Port=5
  PFwF : Inport  Port=6
  PFwR : Inport  Port=7
  BodyFrm : Inport  Port=8
  FxIn : Subsystem  VariantControl=1
  xdotin : Subsystem  VariantControl=0
  PF : Outport  VectorParamsAs1DForOutWhenUnconnected=off
  PM : Outport  Port=2  VectorParamsAs1DForOutWhenUnconnected=off
  ax : Outport  Port=3  VectorParamsAs1DForOutWhenUnconnected=off

== system sim_aut_dual_scen/vehicle/dual-track/Vehicle Body 3DOF Dual Track/Signal Routing/Signal Routing/Power/xdot mode/FxIn ==
  PFExt : Inport
  PMExt : Inport  Port=2
  PFh : Inport  Port=3
  PMh : Inport  Port=4
  PFDrag : Inport  Port=5
  PFwF : Inport  Port=6
  PFwR : Inport  Port=7
  BodyFrm : Inport  Port=8
  Bus Selector2 : BusSelector  OutputSignals=Cg.Acc.ax
  Selector1 : Selector  InputPortWidth=3  IndexOptions=Index vector (dialog)  Indices=[1 2]  OutputSizes=1
  Selector2 : Selector  InputPortWidth=3  IndexOptions=Index vector (dialog)  Indices=[3]  OutputSizes=1
  Selector3 : Selector  InputPortWidth=3  IndexOptions=Index vector (dialog)  Indices=[3]  OutputSizes=1
  Selector4 : Selector  InputPortWidth=3  IndexOptions=Index vector (dialog)  Indices=[1 2]  OutputSizes=1
  Sum : Sum  Inputs=|++
  Sum1 : Sum  Inputs=|++
  Terminator : Terminator
  Terminator2 : Terminator
  Terminator3 : Terminator
  PF : Outport  VectorParamsAs1DForOutWhenUnconnected=off
  PM : Outport  Port=2  VectorParamsAs1DForOutWhenUnconnected=off
  ax : Outport  Port=3  VectorParamsAs1DForOutWhenUnconnected=off
  wires:
  Sum1/1 -> PF/1
  Selector4/1 -> Sum1/2
  PFh/1 -> Selector4/1
  Selector2/1 -> Sum/2
  Sum/1 -> PM/1
  PMh/1 -> Selector2/1
  PFExt/1 -> Selector1/1
  PMExt/1 -> Selector3/1
  PFDrag/1 -> Terminator/1
  Selector3/1 -> Sum/1
  Selector1/1 -> Sum1/1
  PFwR/1 -> Terminator3/1
  PFwF/1 -> Terminator2/1
  BodyFrm/1 -> Bus Selector2/1
  Bus Selector2/1 -> ax/1  "<ax>"

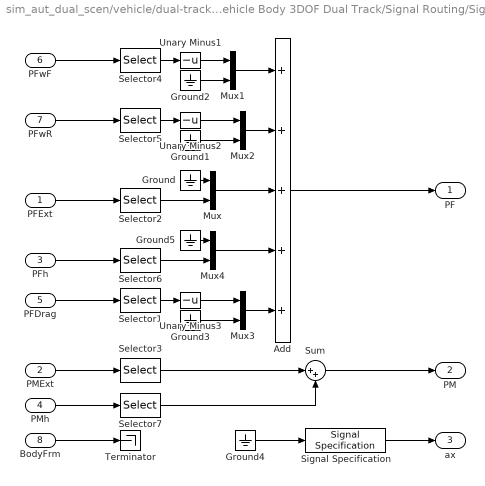
== system sim_aut_dual_scen/vehicle/dual-track/Vehicle Body 3DOF Dual Track/Signal Routing/Signal Routing/Power/xdot mode/xdotin ==
  PFExt : Inport
  PMExt : Inport  Port=2
  PFh : Inport  Port=3
  PMh : Inport  Port=4
  PFDrag : Inport  Port=5
  PFwF : Inport  Port=6
  PFwR : Inport  Port=7
  BodyFrm : Inport  Port=8
  Add : Sum  Inputs=+++++
  Ground{,1..5} (6 alike) : Ground
  Mux{,1..4} (5 alike) : Mux  Inputs=2
  Selector1 : Selector  InputPortWidth=3  IndexOptions=Index vector (dialog)  Indices=[1]  OutputSizes=1
  Selector2 : Selector  InputPortWidth=3  IndexOptions=Index vector (dialog)  Indices=[2]  OutputSizes=1
  Selector3 : Selector  InputPortWidth=3  IndexOptions=Index vector (dialog)  Indices=[3]  OutputSizes=1
  Selector4 : Selector  InputPortWidth=3  IndexOptions=Index vector (dialog)  Indices=[1]  OutputSizes=1
  Selector5 : Selector  InputPortWidth=3  IndexOptions=Index vector (dialog)  Indices=[1]  OutputSizes=1
  Selector6 : Selector  InputPortWidth=3  IndexOptions=Index vector (dialog)  Indices=[2]  OutputSizes=1
  Selector7 : Selector  InputPortWidth=3  IndexOptions=Index vector (dialog)  Indices=[3]  OutputSizes=1
  Signal Specification : SignalSpecification  Unit=gn
  Sum : Sum  Inputs=|++
  Terminator : Terminator
  Unary Minus1 : UnaryMinus
  Unary Minus2 : UnaryMinus
  Unary Minus3 : UnaryMinus
  PF : Outport  VectorParamsAs1DForOutWhenUnconnected=off
  PM : Outport  Port=2  VectorParamsAs1DForOutWhenUnconnected=off
  ax : Outport  Port=3  VectorParamsAs1DForOutWhenUnconnected=off
  wires:
  Selector7/1 -> Sum/2
  Sum/1 -> PM/1
  PMh/1 -> Selector7/1
  PFh/1 -> Selector6/1
  Mux4/1 -> Add/4
  Ground5/1 -> Mux4/1
  Selector6/1 -> Mux4/2
  Add/1 -> PF/1
  PMExt/1 -> Selector3/1
  PFExt/1 -> Selector2/1
  PFDrag/1 -> Selector1/1
  Selector1/1 -> Unary Minus3/1
  Selector2/1 -> Mux/2
  Ground/1 -> Mux/1
  Mux/1 -> Add/3
  PFwF/1 -> Selector4/1
  PFwR/1 -> Selector5/1
  Ground1/1 -> Mux2/2
  Selector4/1 -> Unary Minus1/1
  Ground2/1 -> Mux1/2
  Selector5/1 -> Unary Minus2/1
  Mux2/1 -> Add/2
  Mux1/1 -> Add/1
  Unary Minus1/1 -> Mux1/1
  Unary Minus2/1 -> Mux2/1
  Ground3/1 -> Mux3/2
  Mux3/1 -> Add/5
  Selector3/1 -> Sum/1
  Unary Minus3/1 -> Mux3/1
  BodyFrm/1 -> Terminator/1
  Ground4/1 -> Signal Specification/1
  Signal Specification/1 -> ax/1

== system sim_aut_dual_scen/vehicle/dual-track/Vehicle Body 3DOF Dual Track/Signal Routing/Signal Routing/state2bus/Angle Wrap/None ==
  u : Inport
  y : Outport  VectorParamsAs1DForOutWhenUnconnected=off
  wires:
  u/1 -> y/1

== system sim_aut_dual_scen/vehicle/dual-track/Vehicle Body 3DOF Dual Track/Signal Routing/Signal Routing/state2bus/xddot2ax/m^22gn ==
  ay : Inport  Unit=m/s^2
  ax : Inport  Port=2  Unit=m/s^2
  Unit Conversion : UnitConversion
  Unit Conversion1 : UnitConversion
  ay_g : Outport  Unit=gn  VectorParamsAs1DForOutWhenUnconnected=off
  ax_g : Outport  Port=2  Unit=gn  VectorParamsAs1DForOutWhenUnconnected=off
  wires:
  Unit Conversion1/1 -> ax_g/1
  Unit Conversion/1 -> ay_g/1
  ax/1 -> Unit Conversion1/1
  ay/1 -> Unit Conversion/1

== system sim_aut_dual_scen/vehicle/dual-track/Vehicle Body 3DOF Dual Track/Signal Routing/Signal Routing Dual/Power/xdot mode/FxIn ==
  PFExt : Inport
  PMExt : Inport  Port=2
  PFh : Inport  Port=3
  PMh : Inport  Port=4
  PFDrag : Inport  Port=5
  PFwF : Inport  Port=6
  PFwR : Inport  Port=7
  BodyFrm : Inport  Port=8
  Bus Selector2 : BusSelector  OutputSignals=Cg.Acc.ax
  Selector1 : Selector  InputPortWidth=3  IndexOptions=Index vector (dialog)  Indices=[1 2]  OutputSizes=1
  Selector2 : Selector  InputPortWidth=3  IndexOptions=Index vector (dialog)  Indices=[3]  OutputSizes=1
  Selector3 : Selector  InputPortWidth=3  IndexOptions=Index vector (dialog)  Indices=[3]  OutputSizes=1
  Selector4 : Selector  InputPortWidth=3  IndexOptions=Index vector (dialog)  Indices=[1 2]  OutputSizes=1
  Sum : Sum  Inputs=|++
  Sum1 : Sum  Inputs=|++
  Terminator : Terminator
  Terminator2 : Terminator
  Terminator3 : Terminator
  PF : Outport  VectorParamsAs1DForOutWhenUnconnected=off
  PM : Outport  Port=2  VectorParamsAs1DForOutWhenUnconnected=off
  ax : Outport  Port=3  VectorParamsAs1DForOutWhenUnconnected=off
  wires:
  Sum1/1 -> PF/1
  Selector4/1 -> Sum1/2
  PFh/1 -> Selector4/1
  Sum/1 -> PM/1
  Selector2/1 -> Sum/2
  PMh/1 -> Selector2/1
  PFExt/1 -> Selector1/1
  PMExt/1 -> Selector3/1
  PFDrag/1 -> Terminator/1
  Selector3/1 -> Sum/1
  Selector1/1 -> Sum1/1
  PFwR/1 -> Terminator3/1
  PFwF/1 -> Terminator2/1
  BodyFrm/1 -> Bus Selector2/1
  Bus Selector2/1 -> ax/1  "<ax>"

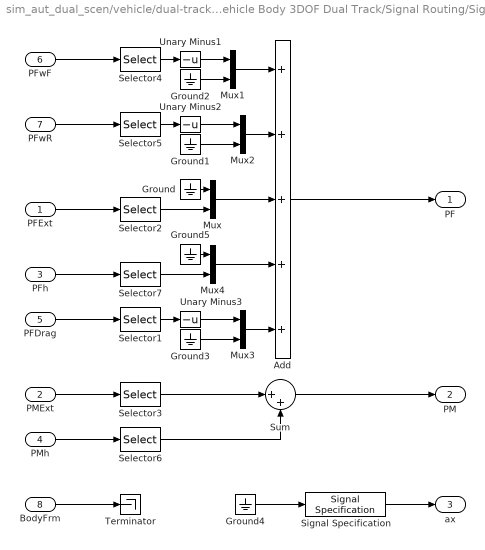
== system sim_aut_dual_scen/vehicle/dual-track/Vehicle Body 3DOF Dual Track/Signal Routing/Signal Routing Dual/Power/xdot mode/xdotin ==
  PFExt : Inport
  PMExt : Inport  Port=2
  PFh : Inport  Port=3
  PMh : Inport  Port=4
  PFDrag : Inport  Port=5
  PFwF : Inport  Port=6
  PFwR : Inport  Port=7
  BodyFrm : Inport  Port=8
  Add : Sum  Inputs=+++++
  Ground{,1..5} (6 alike) : Ground
  Mux{,1..4} (5 alike) : Mux  Inputs=2
  Selector1 : Selector  InputPortWidth=3  IndexOptions=Index vector (dialog)  Indices=[1]  OutputSizes=1
  Selector2 : Selector  InputPortWidth=3  IndexOptions=Index vector (dialog)  Indices=[2]  OutputSizes=1
  Selector3 : Selector  InputPortWidth=3  IndexOptions=Index vector (dialog)  Indices=[3]  OutputSizes=1
  Selector4 : Selector  InputPortWidth=3  IndexOptions=Index vector (dialog)  Indices=[1]  OutputSizes=1
  Selector5 : Selector  InputPortWidth=3  IndexOptions=Index vector (dialog)  Indices=[1]  OutputSizes=1
  Selector6 : Selector  InputPortWidth=3  IndexOptions=Index vector (dialog)  Indices=[3]  OutputSizes=1
  Selector7 : Selector  InputPortWidth=3  IndexOptions=Index vector (dialog)  Indices=[2]  OutputSizes=1
  Signal Specification : SignalSpecification  Unit=gn
  Sum : Sum  Inputs=|++
  Terminator : Terminator
  Unary Minus1 : UnaryMinus
  Unary Minus2 : UnaryMinus
  Unary Minus3 : UnaryMinus
  PF : Outport  VectorParamsAs1DForOutWhenUnconnected=off
  PM : Outport  Port=2  VectorParamsAs1DForOutWhenUnconnected=off
  ax : Outport  Port=3  VectorParamsAs1DForOutWhenUnconnected=off
  wires:
  Mux4/1 -> Add/4
  Ground5/1 -> Mux4/1
  Selector7/1 -> Mux4/2
  PFh/1 -> Selector7/1
  Selector6/1 -> Sum/2
  Sum/1 -> PM/1
  PMh/1 -> Selector6/1
  Add/1 -> PF/1
  PMExt/1 -> Selector3/1
  PFExt/1 -> Selector2/1
  PFDrag/1 -> Selector1/1
  Selector1/1 -> Unary Minus3/1
  Selector2/1 -> Mux/2
  Ground/1 -> Mux/1
  Mux/1 -> Add/3
  PFwF/1 -> Selector4/1
  PFwR/1 -> Selector5/1
  Ground1/1 -> Mux2/2
  Selector4/1 -> Unary Minus1/1
  Ground2/1 -> Mux1/2
  Selector5/1 -> Unary Minus2/1
  Mux2/1 -> Add/2
  Mux1/1 -> Add/1
  Unary Minus1/1 -> Mux1/1
  Unary Minus2/1 -> Mux2/1
  Ground3/1 -> Mux3/2
  Mux3/1 -> Add/5
  Selector3/1 -> Sum/1
  Unary Minus3/1 -> Mux3/1
  BodyFrm/1 -> Terminator/1
  Ground4/1 -> Signal Specification/1
  Signal Specification/1 -> ax/1

== matlab function sim_aut_dual_scen/vehicle/dual-track/Vehicle Body 3DOF Dual Track/vehicle model ==
  data: delta_f input; delta_r input; mu input; a parameter; b parameter; h parameter; d parameter; w parameter; m parameter; NF parameter; NR parameter; Izz parameter; g parameter; Fxtire_sat parameter size=1; Fytire_sat parameter size=1; trackMode parameter; inputMode parameter; xdot_tol parameter; Fznom parameter size=1; F_f input; F_r input; F_ext input size=3; M_ext input size=3; Fh input size=3; Mh input size=3; Cy_f input; Cy_r input; dh input; hl input; hh input; yOut output size=3; FBody output size=3; MBody output size=3; FOut output; FTire output; Fg output size=3; wheelInfo output; stateDer output size=4; stateVec input size=4; status output size=1
function [yOut,FBody,MBody,FOut,FTire,Fg,wheelInfo,stateDer,status] = fcn(delta_f,delta_r,mu,a,b,h,d,w,m,NF,NR,Izz,g,Fxtire_sat,Fytire_sat,trackMode,inputMode,xdot_tol,Fznom,F_f,F_r,F_ext,M_ext,Fh,Mh,Cy_f,Cy_r,dh,hl,hh,stateVec)%#codegen
coder.allowpcode('plain')
switch trackMode
    case 1
       [yOut,FBody,MBody,FOut,FTire,Fg,wheelInfo,stateDer,status] = automlvehdynbicycle(delta_f,delta_r,mu,a,b,h,m,NF,NR,Izz,g,Fxtire_sat,Fytire_sat,inputMode,xdot_tol,Fznom,F_f,F_r,F_ext,M_ext,Fh,Mh,Cy_f,Cy_r,dh,hh,stateVec);
    case 2
       [yOut,FBody,MBody,FOut,FTire,Fg,wheelInfo,stateDer,status] = automlvehdyndualtrack(delta_f,delta_r,mu,a,b,h,d,w,m,NF,NR,Izz,g,Fxtire_sat,Fytire_sat,inputMode,xdot_tol,Fznom,F_f,F_r,F_ext,M_ext,Fh,Mh,Cy_f,Cy_r,dh,hl,hh,stateVec);
end
end

== matlab function sim_aut_dual_scen/road scenario/MATLAB Function1 ==
  data: ze input; egoPose output Bus: ActorPose
function egoPose = createPose(ze)

egoPose.ActorID = uint32(1);

egoPose.Position = [ze(1) ze(2) 0];

egoPose.Velocity = [ze(4) ze(5) 0];

egoPose.Roll  = 0;
egoPose.Pitch = 0;
egoPose.Yaw   = ze(3)*180/pi;
egoPose.AngularVelocity = [0 0 ze(6)*180/pi];

== matlab function sim_aut_dual_scen/reference generator1/MATLAB Function1 ==
  data: Np input; ref output; ref_tr input; ze input; ref_pose output
function [ref,ref_pose] =ref_gen(Np,ref_tr,ze)

% Point of the reference trajectory closest to the vehicle.
N=size(ref_tr,1);
dis=vecnorm(ref_tr(:,1:2)'-ze(1:2)*ones(1,N));
[~,c]=min(dis);
ref_pose=ref_tr(c,:)';

% Portion of the reference trajectory corresponding to
% the time interval [t t+Tp] at the speed vx_ref.
NS=50;
ir=round(linspace(c,c+Np-1,NS+1));

ref0=[ref_tr(ir(1:NS),1:2)';zeros(1,NS)];
ref=reshape(ref0,3*NS,1);

== matlab function sim_aut_dual_scen/reference generator1/Subsystem/MATLAB Function2 ==
  data: ref_pose input; e_ct output; ze input; e_h output
function [e_ct,e_h]=errors(ref_pose,ze)

pose_f=ze(1:3);

% Wrap angles in the interval [0,2*pi]
ref_pose(3)=wrap_to_2pi(ref_pose(3));
pose_f(3)=wrap_to_2pi(pose_f(3));

% Cross-track error  
d=ref_pose(1:2)-pose_f(1:2);
e_ct=d(2)*cos(ref_pose(3))-d(1)*sin(ref_pose(3));

% Heading error
e_h=wrap_to_pi(ref_pose(3)-pose_f(3));

end

%--------------------------------------------------------------------------

function lambda = wrap_to_2pi(lambda)
%   Wraps angle in radians to [0 2*pi]
%   lambdaWrapped = wrapTo2Pi(LAMBDA) wraps angles in LAMBDA, in radians,
%   to the interval [0 2*pi] such that zero maps to zero and 2*pi maps
%   to 2*pi. (In general, positive multiples of 2*pi map to 2*pi and
%   negative multiples of 2*pi map to zero.)
%   See also wrapToPi, wrapTo180, wrapTo360.
positiveInput = (lambda > 0);
lambda = mod(lambda, 2*pi);
lambda((lambda == 0) & positiveInput) = 2*pi;
end

function lambda = wrap_to_pi(lambda)
%   Wraps angle in radians to [-pi pi]
%   lambdaWrapped = wrapToPi(LAMBDA) wraps angles in LAMBDA, in radians,
%   to the interval [-pi pi] such that pi maps to pi and -pi maps to
%   -pi.  (In general, odd, positive multiples of pi map to pi and odd,
%   negative multiples of pi map to -pi.)
%   See also wrapTo2Pi, wrapTo180, wrapTo360.
q = (lambda < -pi) | (pi < lambda);
lambda(q) = wrap_to_2pi(lambda(q) + pi) - pi;
end
